simulink model "Attitude_Control_System_of_Flying_Vehicle"  (R2016b)
settings: Solver=VariableStepAuto  StartTime=0.0  StopTime=1  MaxStep=0.0001  RelTol=1e-3
settings Model: Creator=Administrator  LastModifiedBy=Administrator

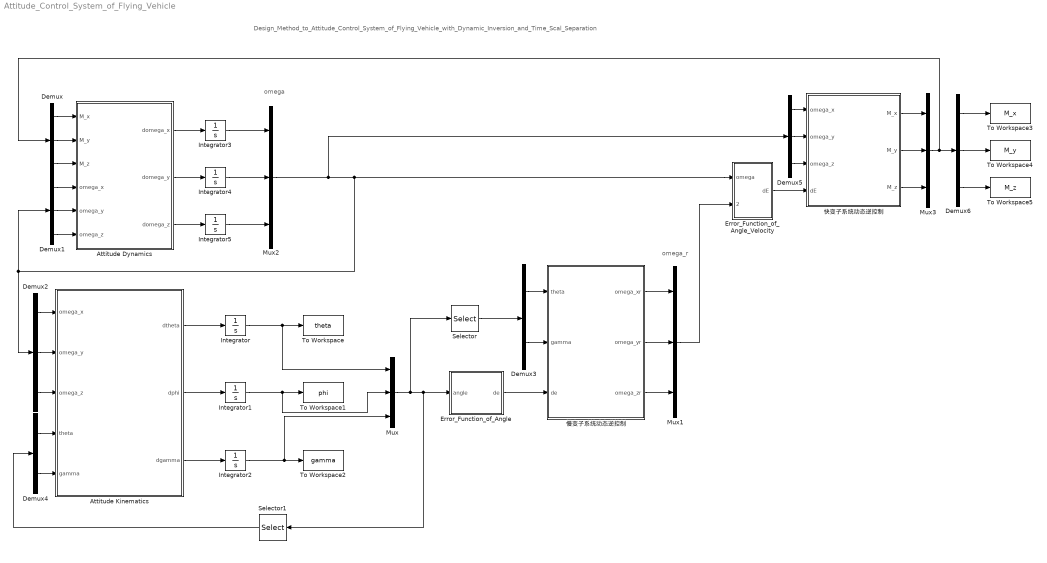
== system Attitude_Control_System_of_Flying_Vehicle ==
  note: omega_r
  note: omega
  note: Design_Method_to_Attitude_Control_System_of_Flying_Vehicle_with_Dynamic_Inversion_and_Time_Scal_Separation
  Attitude Dynamics : MATLAB Function  TreatAsAtomicUnit=on
  Attitude Kinematics : MATLAB Function  TreatAsAtomicUnit=on
  Demux{,1..2,5..6} (5 alike) : Demux  Outputs=3
  Demux3 : Demux  Outputs=2
  Demux4 : Demux  Outputs=2
  Error_Function_of_Angle : Subsystem
  Error_Function_of_Angle_Velocity : Subsystem
  Integrator{,1..5} (6 alike) : Integrator
  Mux{,1..3} (4 alike) : Mux  Inputs=3
  Selector : Selector  InputPortWidth=3  IndexOptions=Index vector (dialog)  Indices=[1 3]  OutputSizes=1
  Selector1 : Selector  InputPortWidth=3  IndexOptions=Index vector (dialog)  Indices=[1 3]  OutputSizes=1
  To Workspace : ToWorkspace  VariableName=theta  SampleTime=-1
  To Workspace1 : ToWorkspace  VariableName=phi  SampleTime=-1
  To Workspace2 : ToWorkspace  VariableName=gamma  SampleTime=-1
  To Workspace3 : ToWorkspace  VariableName=M_x  SampleTime=-1
  To Workspace4 : ToWorkspace  VariableName=M_y  SampleTime=-1
  To Workspace5 : ToWorkspace  VariableName=M_z  SampleTime=-1
  快变子系统动态逆控制 : MATLAB Function  TreatAsAtomicUnit=on
  慢变子系统动态逆控制 : MATLAB Function  TreatAsAtomicUnit=on
  wires:
  Attitude Kinematics/1(dtheta) -> Integrator/1
  Attitude Kinematics/2(dphi) -> Integrator1/1
  Attitude Kinematics/3(dgamma) -> Integrator2/1
  Integrator/1 -> Mux/1, To Workspace/1
  Integrator1/1 -> Mux/2, To Workspace1/1
  Integrator2/1 -> Mux/3, To Workspace2/1
  Mux/1 -> Selector/1, Selector1/1, Error_Function_of_Angle/1(angle)
  Error_Function_of_Angle/1(de) -> 慢变子系统动态逆控制/3(de)
  Attitude Dynamics/1(domega_x) -> Integrator3/1
  Attitude Dynamics/2(domega_y) -> Integrator4/1
  Attitude Dynamics/3(domega_z) -> Integrator5/1
  Integrator3/1 -> Mux2/1
  Integrator4/1 -> Mux2/2
  Integrator5/1 -> Mux2/3
  慢变子系统动态逆控制/1(omega_xr) -> Mux1/1
  慢变子系统动态逆控制/2(omega_yr) -> Mux1/2
  慢变子系统动态逆控制/3(omega_zr) -> Mux1/3
  Mux2/1 -> Demux5/1, Demux2/1, Demux1/1, Error_Function_of_Angle_Velocity/1(omega)
  Mux1/1 -> Error_Function_of_Angle_Velocity/2(omega_r)
  Error_Function_of_Angle_Velocity/1(dE) -> 快变子系统动态逆控制/4(dE)
  快变子系统动态逆控制/1(M_x) -> Mux3/1
  快变子系统动态逆控制/2(M_y) -> Mux3/2
  Demux/1 -> Attitude Dynamics/1(M_x)
  Demux/2 -> Attitude Dynamics/2(M_y)
  Demux/3 -> Attitude Dynamics/3(M_z)
  Mux3/1 -> Demux6/1, Demux/1
  Demux1/1 -> Attitude Dynamics/4(omega_x)
  Demux1/2 -> Attitude Dynamics/5(omega_y)
  Demux1/3 -> Attitude Dynamics/6(omega_z)
  Demux2/1 -> Attitude Kinematics/1(omega_x)
  Demux2/2 -> Attitude Kinematics/2(omega_y)
  Demux2/3 -> Attitude Kinematics/3(omega_z)
  Demux3/1 -> 慢变子系统动态逆控制/1(theta)
  Demux3/2 -> 慢变子系统动态逆控制/2(gamma)
  Selector/1 -> Demux3/1
  Demux4/1 -> Attitude Kinematics/4(theta)
  Demux4/2 -> Attitude Kinematics/5(gamma)
  Selector1/1 -> Demux4/1
  快变子系统动态逆控制/3(M_z) -> Mux3/3
  Demux5/2 -> 快变子系统动态逆控制/2(omega_y)
  Demux5/1 -> 快变子系统动态逆控制/1(omega_x)
  Demux5/3 -> 快变子系统动态逆控制/3(omega_z)
  Demux6/1 -> To Workspace3/1
  Demux6/2 -> To Workspace4/1
  Demux6/3 -> To Workspace5/1

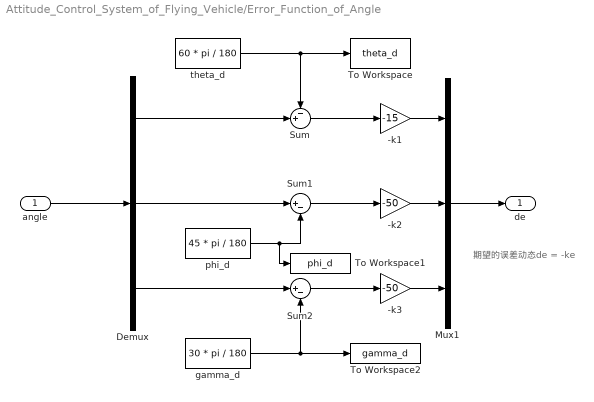
== system Attitude_Control_System_of_Flying_Vehicle/Error_Function_of_Angle ==
  note: 期望的误差动态de = -ke
  angle : Inport
  -k1 : Gain  Gain=-15
  -k2 : Gain  Gain=-50
  -k3 : Gain  Gain=-50
  Demux : Demux  Outputs=3
  Mux1 : Mux  Inputs=3
  Sum : Sum  Inputs=-+|
  Sum1 : Sum  Inputs=|+-
  Sum2 : Sum  Inputs=|+-
  To Workspace : ToWorkspace  VariableName=theta_d  SampleTime=-1
  To Workspace1 : ToWorkspace  VariableName=phi_d  SampleTime=-1
  To Workspace2 : ToWorkspace  VariableName=gamma_d  SampleTime=-1
  gamma_d : Constant  Value=30 * pi / 180
  phi_d : Constant  Value=45 * pi / 180
  theta_d : Constant  Value=60 * pi / 180
  de : Outport
  wires:
  Sum/1 -> -k1/1
  angle/1 -> Demux/1
  Demux/3 -> Sum2/1
  Sum1/1 -> -k2/1
  Sum2/1 -> -k3/1
  theta_d/1 -> To Workspace/1, Sum/1
  phi_d/1 -> To Workspace1/1, Sum1/2
  Demux/1 -> Sum/2
  gamma_d/1 -> To Workspace2/1, Sum2/2
  Demux/2 -> Sum1/1
  Mux1/1 -> de/1
  -k1/1 -> Mux1/1
  -k2/1 -> Mux1/2
  -k3/1 -> Mux1/3

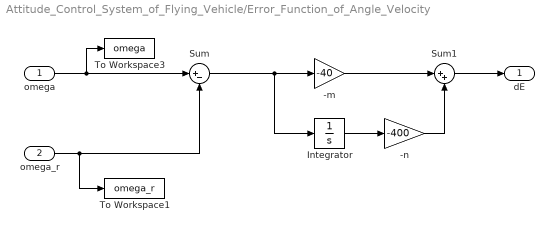
== system Attitude_Control_System_of_Flying_Vehicle/Error_Function_of_Angle_Velocity ==
  omega : Inport
  omega_r : Inport  Port=2
  -m : Gain  Gain=-40
  -n : Gain  Gain=-400
  Integrator : Integrator
  Sum : Sum  Inputs=|+-
  Sum1 : Sum  Inputs=|++
  To Workspace1 : ToWorkspace  VariableName=omega_r  SampleTime=-1
  To Workspace3 : ToWorkspace  VariableName=omega  SampleTime=-1
  dE : Outport
  wires:
  omega/1 -> To Workspace3/1, Sum/1
  omega_r/1 -> To Workspace1/1, Sum/2
  Sum/1 -> Integrator/1, -m/1
  Sum1/1 -> dE/1
  Integrator/1 -> -n/1
  -m/1 -> Sum1/1
  -n/1 -> Sum1/2

== matlab function Attitude_Control_System_of_Flying_Vehicle/Attitude Dynamics ==
  data: M_x input; domega_x output; M_y input; M_z input; omega_x input; omega_y input; omega_z input; domega_y output; domega_z output
%% 姿态动力学方程
function [domega_x,domega_y,domega_z] = fcn(M_x,M_y,M_z,omega_x,omega_y,omega_z)

Jx = 0.1;
Jy = 1;
Jz = 1;

domega_x = 1 / Jx * (M_x - (Jz - Jy) * omega_y * omega_z);
domega_y = 1 / Jy * (M_y - (Jx - Jz) * omega_x * omega_z);
domega_z = 1 / Jz * (M_z - (Jy - Jx) * omega_x * omega_y);

== matlab function Attitude_Control_System_of_Flying_Vehicle/Attitude Kinematics ==
  data: omega_x input; dtheta output; omega_y input; omega_z input; dphi output; dgamma output; theta input; gamma input
%% 姿态运动学方程
function [dtheta,dphi,dgamma] = fcn(omega_x,omega_y,omega_z,theta,gamma)

omega = [omega_x,omega_y,omega_z]';
A = zeros(3,3);

%% 这个矩阵真实坑，初值为0就会使它是个奇异矩阵
% A(1,:) = [0                  sin(gamma)                           cos(gamma)];
% A(2,:) = [0                  cos(gamma) / cos(theta)      -sin(gamma) / cos(theta)];
% A(3,:) = [0                 -tan(theta) * cos(gamma)      tan(theta) * sin(gamma)];
A(1,:) = [0                        sin(theta)                               1]; % 直接使用求逆后的矩阵
A(2,:) = [sin(gamma)       cos(theta) * cos(gamma)       0];
A(3,:) = [cos(gamma)      -cos(theta) * sin(gamma)      0];

dangle = inv(A) * omega;

dtheta     = dangle(1);
dphi        = dangle(2);
dgamma = dangle(3);

== matlab function Attitude_Control_System_of_Flying_Vehicle/慢变子系统动态逆控制 ==
  data: theta input; omega_xr output; omega_yr output; omega_zr output; gamma input; de input
function [omega_xr,omega_yr,omega_zr] = fcn(theta,gamma,de)

R = zeros(3,3);
%% 这样求逆在0初值时矩阵奇异！
% R(1,:) = [0                  sin(gamma)                           cos(gamma)];
% R(2,:) = [0                  cos(gamma) / cos(theta)      -sin(gamma) / cos(theta)];
% R(3,:) = [0                 -tan(theta) * cos(gamma)      tan(theta) * sin(gamma)];
% 
% omega_r = inv(R) * de;
R(1,:) = [0                        sin(theta)                               1]; % 直接使用求逆后的矩阵
R(2,:) = [sin(gamma)       cos(theta) * cos(gamma)       0];
R(3,:) = [cos(gamma)      -cos(theta) * sin(gamma)      0];

omega_r = R * de;

omega_xr = omega_r(1);
omega_yr = omega_r(2);
omega_zr = omega_r(3);

== matlab function Attitude_Control_System_of_Flying_Vehicle/快变子系统动态逆控制 ==
  data: omega_x input; omega_y input; omega_z input; dE input; M_x output; M_y output; M_z output
function [M_x,M_y,M_z] = fcn(omega_x,omega_y,omega_z,dE)

Jx = 0.1;
Jy = 1;
Jz = 1;

J = zeros(3,3);
J(1,1) = 1 / Jx;
J(2,2) = 1 / Jy;
J(3,3) = 1 / Jz;

B = zeros(3,1);
B(1) = dE(1) - (Jy - Jz) / Jx * omega_y *  omega_z;
B(2) = dE(2) - (Jz - Jx) / Jy * omega_x *  omega_z;
B(3) = dE(3) - (Jx - Jy) / Jz * omega_x *  omega_y;

M = inv(J) * B;

M_x = M(1);
M_y = M(2);
M_z = M(3);
